simulink model "project1simulink"  (R2023a)
settings: Solver=VariableStepAuto  StartTime=0.0  StopTime=10.0  RelTol=1e-3
libraries: aerolibanim x1
settings Model: Creator=sushm  LastModifiedBy=sushm

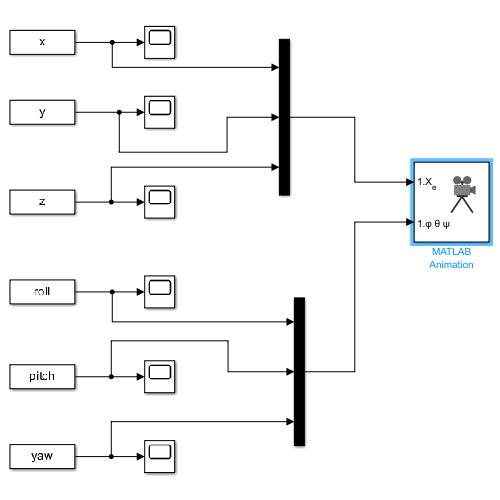
[thumbnail: Simulink's stored preview of the top-level diagram]
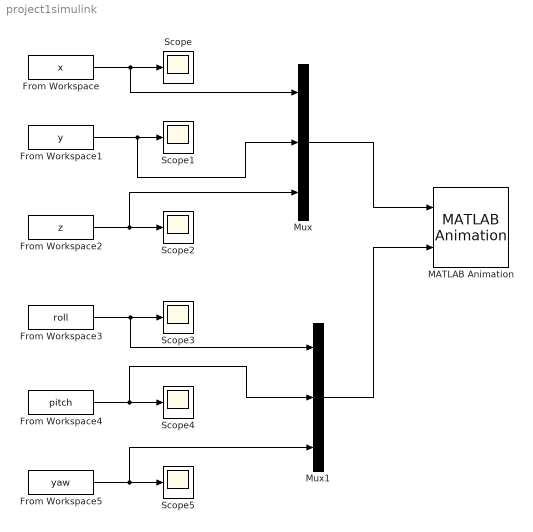
== system project1simulink ==
  From Workspace : FromWorkspace  VariableName=x
  From Workspace1 : FromWorkspace  VariableName=y
  From Workspace2 : FromWorkspace  VariableName=z
  From Workspace3 : FromWorkspace  VariableName=roll
  From Workspace4 : FromWorkspace  VariableName=pitch
  From Workspace5 : FromWorkspace  VariableName=yaw
  MATLAB Animation : aerolibanim/MATLAB Animation  Tag=Matlab Animation 6 DOF  Vehicles=1  Geometries='pa24-250_blue.ac'  BoundingBoxCoordinates=[-100,100,-100,100,-100,100]  CameraOffset=[-150,-50,0]  CameraViewAngle=3  SampleTime=0.01  FigurePosition=[1,49,1536,7.664000e+02]
  Mux : Mux  Inputs=3
  Mux1 : Mux  Inputs=3
  Scope{,1..5} (6 alike) : Scope
  wires:
  From Workspace/1 -> Mux/1, Scope/1
  From Workspace1/1 -> Mux/2, Scope1/1
  From Workspace2/1 -> Mux/3, Scope2/1
  From Workspace3/1 -> Mux1/1, Scope3/1
  From Workspace4/1 -> Mux1/2, Scope4/1
  From Workspace5/1 -> Mux1/3, Scope5/1
  Mux/1 -> MATLAB Animation/1
  Mux1/1 -> MATLAB Animation/2
